simulink model "Ejercicio1"  (R2020a)
settings: Solver=VariableStepAuto  StartTime=0.0  StopTime=40  MaxStep=0.001  RelTol=1e-3
values from neighbouring files (symbols this model uses):
  a = 200    [Ejercicio1_parametros.m]
  alfa = 1    [Ejercicio1_parametros.m]
  alfa_c = 0    [Ejercicio1_parametros.m]
  b = 10000    [Ejercicio1_parametros.m]
  cl = 0    [Ejercicio1_parametros.m]
  g = 9.82    [Ejercicio1_parametros.m]
  kd = k(indice, 2)    [Ejercicio1_parametros.m]
  ki = k(indice, 3)    [Ejercicio1_parametros.m]
  kp = k(indice, 1)    [Ejercicio1_parametros.m]
  m = 1000    [Ejercicio1_parametros.m]
  ol = 1    [Ejercicio1_parametros.m]
undefined symbols (not defined in the file or in its folder): sigbuilder_block
libraries: simulink x1, simulink_extras x1
settings Model: Creator=juan  LastModifiedBy=juan

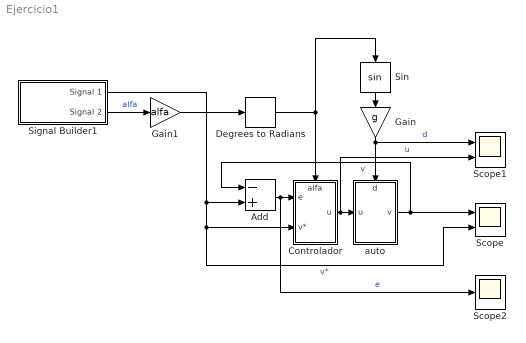
== system Ejercicio1 ==
  Add : Sum  Inputs=-+
  Controlador : Subsystem
      settings: PortSchema="{\"entries\":[{\"content\":{\"sides\":[{\"content\":{\"connectorIds\":[\"In1\",\"In2\"]},\"type\":\"ConnectorPlacement.EquallySpacedRectSide\",\"uuid\":\"eda19091-e346-4b3f-a1d2-cc7b7af4e522\"},{\"content\":{\"connectorIds\":[\"Out1\"],\"side\":\"RIGHT\"},\"type\":\"ConnectorPlacement.EquallySpacedRectSide\",\"uuid\":\"0e82abb1-9334-4f6a-951a-a03f8783b358\"},{\"content\":{\"connectorIds\":[\"In3\"],\"side\":\"TOP\"},\"type\":\"ConnectorPlacement.EquallySpacedRectSide\",\"uuid\":\"7bc2c83a-fea4-452a-a876-fba0fe75db6a\"}]},\"type\":\"ConnectorPlacement.EquallySpacedConnector\",\"uuid\":\"491ee8e8-9af8-40f2-9de4-dd76d60debaf\"}],\"packageUris\":[\"http://schema.mathworks.com/mf0/Connector/19700101\"],\"version\":\"1.0\"}"
  Degrees to Radians : simulink_extras/Transformations/Degrees to Radians
  Gain : Gain  Gain=g
  Gain1 : Gain  Gain=alfa
  Scope : Scope  NumInputPorts=2
  Scope1 : Scope  NumInputPorts=2
  Scope2 : Scope
  Signal Builder1 : Subsystem  Tag=STV Subsys  LoadFcn=sigbuilder_block('load',[0 22.5 1024.5 495.75 ]);  StartFcn=sigbuilder_block('start');  StopFcn=sigbuilder_block('stop');  ClipboardFcn=sigbuilder_block('clipboard');  mask(Sigbuilder block){tuvar=[0:10]}
      mask help: Simulink:masks:SigbuilderBlock_MD
      mask init:
      | if ~strcmp(get_param(bdroot(gcbh),'SimulationStatus'),'stopped') tuvar = sigbuilder_block('maskInit'); end
      settings: CopyFcn=sigbuilder_block('copy');  DeleteFcn=sigbuilder_block('delete');  ModelCloseFcn=sigbuilder_block('modelClose');  PreSaveFcn=sigbuilder_block('preSave');  PauseFcn=sigbuilder_block('pause');  ContinueFcn=sigbuilder_block('continue');  NameChangeFcn=sigbuilder_block('namechange');  OpenFcn=sigbuilder_block('open',[342.75 141.75 550.5 359.25 ]);  CloseFcn=sigbuilder_block('close');
      mask Display: plot(0, 0, 100, 100,[2, 2, 32, 32, 2], [68, 8, 8, 68, 68],[32, 2], [38, 38], [32, 19, 2],[53, 60, 44], [32, 17, 17, 2],[16, 16, 31, 31]);txt = getActiveGroup(gcbh);text(2, 100, txt,'verticalAlignment', 'top');
  Sin : Trigonometry
  auto : Subsystem
      settings: PortSchema="{\"entries\":[{\"content\":{\"sides\":[{\"content\":{\"connectorIds\":[\"In1\"]},\"type\":\"ConnectorPlacement.EquallySpacedRectSide\",\"uuid\":\"eda19091-e346-4b3f-a1d2-cc7b7af4e522\"},{\"content\":{\"connectorIds\":[\"Out1\"],\"side\":\"RIGHT\"},\"type\":\"ConnectorPlacement.EquallySpacedRectSide\",\"uuid\":\"0e82abb1-9334-4f6a-951a-a03f8783b358\"},{\"content\":{\"connectorIds\":[\"In2\"],\"side\":\"TOP\"},\"type\":\"ConnectorPlacement.EquallySpacedRectSide\",\"uuid\":\"7bc2c83a-fea4-452a-a876-fba0fe75db6a\"}]},\"type\":\"ConnectorPlacement.EquallySpacedConnector\",\"uuid\":\"491ee8e8-9af8-40f2-9de4-dd76d60debaf\"}],\"packageUris\":[\"http://schema.mathworks.com/mf0/Connector/19700101\"],\"version\":\"1.0\"}"
  wires:
  Signal Builder1/1(Signal 1) -> Controlador/2(v*), Scope/2, Add/2  "v*"
  Degrees to Radians/1 -> Sin/1, Controlador/3(alfa)
  Signal Builder1/2(Signal 2) -> Gain1/1  "alfa"
  Controlador/1(u) -> Scope1/2, auto/1(u)  "u"
  Gain/1 -> auto/2(d), Scope1/1  "d"
  Sin/1 -> Gain/1
  auto/1(v) -> Add/1, Scope/1  "v"
  Add/1 -> Scope2/1, Controlador/1(e)  "e"
  Gain1/1 -> Degrees to Radians/1

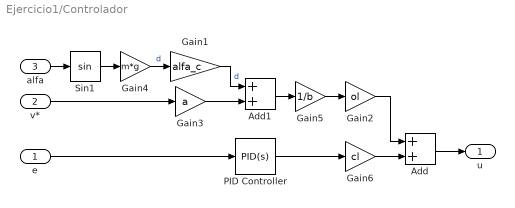
== system Ejercicio1/Controlador ==
  e : Inport
  v* : Inport  Port=2
  alfa : Inport  Port=3
  Add : Sum
  Add1 : Sum
  Gain1 : Gain  Gain=alfa_c
  Gain2 : Gain  Gain=ol
  Gain3 : Gain  Gain=a
  Gain4 : Gain  Gain=m*g
  Gain5 : Gain  Gain=1/b
  Gain6 : Gain  Gain=cl
  PID Controller : simulink/Continuous/PID Controller  Controller=PID  Form=Parallel  TimeDomain=Continuous-time  UseExternalTs=off  SampleTime=-1  IntegratorMethod=Forward Euler  FilterMethod=Forward Euler  ControllerParametersSource=internal  P=kp  I=ki  D=kd  UseFilter=on  N=200  TunerSelectOption=Transfer Function Based (PID Tuner App)  InitialConditionSource=internal  InitialConditionForIntegrator=0  InitialConditionForFilter=0  DifferentiatorICPrevScaledInput=0  ExternalReset=none  TrackingMode=off  Kt=1  LimitOutput=off  UpperSaturationLimit=inf  LowerSaturationLimit=-inf  LinearizeAsGain=on  AntiWindupMode=none  Kb=1  POutMin=[]  POutMax=[]  IOutMin=[]  IOutMax=[]  DOutMin=[]  DOutMax=[]  NOutMin=[]  NOutMax=[]  SumOutMin=[]  SumOutMax=[]  SaturationOutMin=[]  SaturationOutMax=[]  PParamMin=[]  PParamMax=[]  IParamMin=[]  IParamMax=[]  DParamMin=[]  DParamMax=[]  NParamMin=[]  NParamMax=[]  KbParamMin=[]  KbParamMax=[]  KtParamMin=[]  KtParamMax=[]  KbOutMin=[]  KbOutMax=[]  KtOutMin=[]  KtOutMax=[]  IntegratorOutMin=[]  IntegratorOutMax=[]  FilterOutMin=[]  FilterOutMax=[]  SumI1OutMin=[]  SumI1OutMax=[]  SumI2OutMin=[]  SumI2OutMax=[]  SumI3OutMin=[]  SumI3OutMax=[]  SumI4OutMin=[]  SumI4OutMax=[]  SumDOutMin=[]  SumDOutMax=[]  DifferentiatorOutMin=[]  DifferentiatorOutMax=[]  FilterDiffOutCoefMin=[]  FilterDiffOutCoefMax=[]  ReciprocalOutMin=[]  ReciprocalOutMax=[]  SumDenOutMin=[]  SumDenOutMax=[]  SumNumOutMin=[]  SumNumOutMax=[]  DivideOutMin=[]  DivideOutMax=[]  UdiffTsProdOutMin=[]  UdiffTsProdOutMax=[]  NTsProdOutMin=[]  NTsProdOutMax=[]  UintegralTsProdOutMin=[]  UintegralTsProdOutMax=[]  UngainTsProdOutMin=[]  UngainTsProdOutMax=[]  IntegratorContinuousStateAttributes=''  IntegratorStateMustResolveToSignalObject=off  IntegratorRTWStateStorageClass=Auto  FilterContinuousStateAttributes=''  FilterStateMustResolveToSignalObject=off  FilterRTWStateStorageClass=Auto  ParallelPVariant=InternalParameters  IdealPVariant=Disabled  IVariant=InternalParameters  DVariant=InternalParameters  IntegratorVariant=Continuous  SatVariant=Disabled  AWVariant=Passthrough  PCopyVariant=Disabled  TRVariant=Disabled  FdbkBlocksVariant=Forward  IdealPFdbkVariant=Disabled  SatFdbkVariant=Disabled  DerivativeFilterVariant=ContFilter  NVariant=InternalParameters  NCopyVariant=Disabled  FilterICVariant=InternalICsFilter  IntegratorICVariant=InternalICs  ExternalResetVariant=Disabled  TRSumVariant=Passthrough  SumFdbkVariant=Disabled  SumVariant=Sum_PID  TsampFilterVariant=InternalTs  TsampNgainVariant=Passthrough  TsampIntegralVariant=Passthrough
  Sin1 : Trigonometry
  u : Outport
  wires:
  Gain3/1 -> Add1/2
  Gain4/1 -> Gain1/1  "d"
  Add1/1 -> Gain5/1
  Gain5/1 -> Gain2/1
  Sin1/1 -> Gain4/1
  alfa/1 -> Sin1/1
  v*/1 -> Gain3/1
  Gain1/1 -> Add1/1  "d"
  e/1 -> PID Controller/1
  Gain2/1 -> Add/1
  Add/1 -> u/1
  Gain6/1 -> Add/2
  PID Controller/1 -> Gain6/1

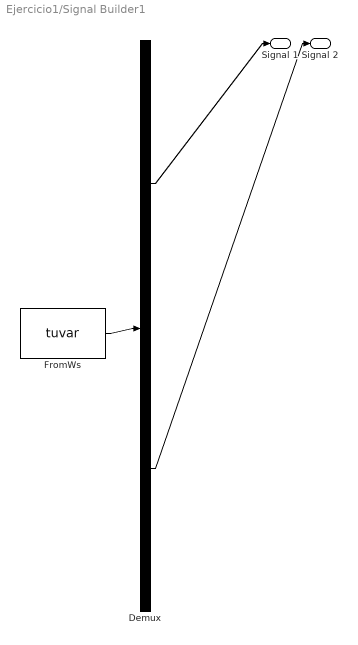
== system Ejercicio1/Signal Builder1 ==
  Demux : Demux  Tag=STV Demux  Outputs=2
      settings: DisplayOption=none
  FromWs : FromWorkspace  Tag=STV FromWs  VariableName=tuvar
      SigBuilderData=|
      | common.afterFinalStr = 'Extrapolate'
      | common.sampleTime = 0
      | dataSet.timeRange = [0 30]
      | dataSet.name = 'Group 1'
      | sbobj.Groups.Name = 'Group 1'
      | sbobj.Groups.Signals(1).Name = 'Signal 1'
      | sbobj.Groups.Signals(1).XData = [0 10 10 30]
      | sbobj.Groups.Signals(1).YData = [25 25 30 30]
      | sbobj.Groups.Signals(2).Name = 'Signal 2'
      | sbobj.Groups.Signals(2).XData = [0 20 20 30]
      | sbobj.Groups.Signals(2).YData = [0 0 2 2]
      | sbobj.Groups.TimeRange = [0 30]
  Signal 1 : Outport  Tag=STV Outport
  Signal 2 : Outport  Tag=STV Outport  Port=2
  wires:
  Demux/1 -> Signal 1/1
  Demux/2 -> Signal 2/1
  FromWs/1 -> Demux/1

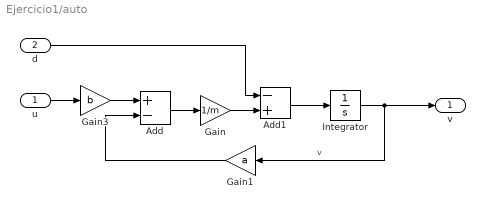
== system Ejercicio1/auto ==
  u : Inport
  d : Inport  Port=2
  Add : Sum  Inputs=+-
  Add1 : Sum  Inputs=-+
  Gain : Gain  Gain=1/m
  Gain1 : Gain  Gain=a
  Gain3 : Gain  Gain=b
  Integrator : Integrator
  v : Outport
  wires:
  Add/1 -> Gain/1
  Gain3/1 -> Add/1
  Gain1/1 -> Add/2
  Integrator/1 -> v/1, Gain1/1  "v"
  u/1 -> Gain3/1
  Add1/1 -> Integrator/1
  Gain/1 -> Add1/2
  d/1 -> Add1/1
